simulink model "PSB_FPGAdesign8_model"  (R2021a)
settings: Solver=VariableStepAuto  StartTime=0.0  StopTime=3000  RelTol=1e-3
values from neighbouring files (symbols this model uses):
  n_channel = 1024    [PSB3_0_script.m]    (also in PSB_FPGAdesign8_script.m)
  parallel_factor = 4    [PSB3_0_script.m]    (also in PSB_FPGAdesign8_script.m)
libraries: xbsIndex_r4 x1089, xrbsSSR_Library x150, dspsrcs4 x48
(part 3 of 7)

== system PSB_FPGAdesign8_model/Baseband_odd_3 ==
  tvalid : Inport
  addr_r : Inport  Port=2
  addr_w : Inport  Port=3
  init_im_odd : Inport  Port=4
  init_re_odd : Inport  Port=5
  dphi_odd : Inport  Port=6
  we : Inport  Port=7
  AddSub1 : xbsIndex_r4/AddSub  mode=Addition  use_carryin=off  use_carryout=off  en=off  latency=2  precision=User Defined  arith_type=Unsigned  n_bits=16  bin_pt=0  quantization=Truncate  overflow=Wrap  use_behavioral_HDL=off  hw_selection=Fabric  pipelined=off  dbl_ovrd=off  block_type=addsub
  CORDIC 6.0 odd_1 : xbsIndex_r4/CORDIC 6.0   functional_selection=Rotate  architectural_configuration=Parallel  pipelining_mode=Optimal  data_format=SignedFraction  phase_format=Scaled_Radians  input_width=18  output_width=16  round_mode=Nearest_Even  iterations=16  precision=20  compensation_scaling=LUT_based  coarse_rotation=on  aclken=off  aresetn=off  out_tready=off  cartesian_has_tuser=off  cartesian_has_tlast=off  cartesian_tuser_width=1  phase_has_tuser=off  phase_has_tlast=off  phase_tuser_width=1  out_tlast_behv=Null  flow_control=NonBlocking  optimize_goal=Resources  trim_axipin_name=on  simulation_type=hybrid_sim  simulation_model=sysgen:cordic_v6_0  data_path_portlist={'s_axis_cartesian_tdata_imag', 's_axis_cartesian_tdata_real', 's_axis_phase_tdata_phase', 'm_axis_dout_tdata_imag', 'm_axis_dout_tdata_real', 'm_axis_dout_tdata_phase','m_axis_dout_tdata'}  ip_name=CORDIC  ip_version=6.0  dsptool_ready=true  ipcore_usecache=true  ipcore_useipmodelcache=true  wrapper_available=true  port_translation_map={ 'aclken' => 'en', 'aresetn' => 'rst' }  block_type=cordic_v6_0
      settings: infoedit=CORDIC 6.0
  Constant10 : xbsIndex_r4/Constant  const=0  gui_display_data_type=Fixed-point  arith_type=Signed (2's comp)  n_bits=18  bin_pt=16  preci_type=Single  exp_width=8  frac_width=24  explicit_period=on  period=1  equ=P=C  opselect=C  inp2=PCIN>>17  opr=+  inp1=P  carry=CIN  dbl_ovrd=off  block_type=constant
  Constant11 : xbsIndex_r4/Constant  const=1  gui_display_data_type=Boolean  arith_type=Boolean  n_bits=16  bin_pt=14  preci_type=Single  exp_width=8  frac_width=24  explicit_period=on  period=1  equ=P=C  opselect=C  inp2=PCIN>>17  opr=+  inp1=P  carry=CIN  dbl_ovrd=off  block_type=constant
  Constant12 : xbsIndex_r4/Constant  const=0  gui_display_data_type=Fixed-point  arith_type=Signed (2's comp)  n_bits=18  bin_pt=16  preci_type=Single  exp_width=8  frac_width=24  explicit_period=on  period=1  equ=P=C  opselect=C  inp2=PCIN>>17  opr=+  inp1=P  carry=CIN  dbl_ovrd=off  block_type=constant
  Constant13 : xbsIndex_r4/Constant  const=0  gui_display_data_type=Fixed-point  arith_type=Unsigned  n_bits=16  bin_pt=0  preci_type=Single  exp_width=8  frac_width=24  explicit_period=on  period=1  equ=P=C  opselect=C  inp2=PCIN>>17  opr=+  inp1=P  carry=CIN  dbl_ovrd=off  block_type=constant
  Constant4 : xbsIndex_r4/Constant  const=0  gui_display_data_type=Boolean  arith_type=Boolean  n_bits=16  bin_pt=14  preci_type=Single  exp_width=8  frac_width=24  explicit_period=on  period=1  equ=P=C  opselect=C  inp2=PCIN>>17  opr=+  inp1=P  carry=CIN  dbl_ovrd=off  block_type=constant
  Constant5 : xbsIndex_r4/Constant  const=0  gui_display_data_type=Boolean  arith_type=Boolean  n_bits=16  bin_pt=14  preci_type=Single  exp_width=8  frac_width=24  explicit_period=on  period=1  equ=P=C  opselect=C  inp2=PCIN>>17  opr=+  inp1=P  carry=CIN  dbl_ovrd=off  block_type=constant
  Constant9 : xbsIndex_r4/Constant  const=0  gui_display_data_type=Boolean  arith_type=Boolean  n_bits=16  bin_pt=14  preci_type=Single  exp_width=8  frac_width=24  explicit_period=on  period=1  equ=P=C  opselect=C  inp2=PCIN>>17  opr=+  inp1=P  carry=CIN  dbl_ovrd=off  block_type=constant
  Convert1 : xbsIndex_r4/Convert  gui_display_data_type=Fixed-point  arith_type="Signed  (2's comp)"  n_bits=18  bin_pt=15  float_type=Single  exp_bits=8  fraction_bits=24  quantization=Truncate  overflow=Wrap  en=off  latency=0  pipeline=off  dbl_ovrd=off  block_type=convert
  DPRAM_dphi_odd_3 : xbsIndex_r4/Dual Port RAM  depth=n_channel/parallel_factor  initVector=dphi_uint16_odd_3  distributed_mem=Block RAM  init_a=0  init_b=0  rst_a=off  rst_b=off  en_a=off  en_b=off  latency=1  write_mode_A=Read Before Write  write_mode_B=Read Before Write  optimize=Area  dbl_ovrd=off  simulation_type=fast_sim  block_type=dpram
  DPRAM_init_im_odd_3 : xbsIndex_r4/Dual Port RAM  depth=n_channel/parallel_factor  initVector=init_im_odd_3  distributed_mem=Block RAM  init_a=0  init_b=0  rst_a=off  rst_b=off  en_a=off  en_b=off  latency=1  write_mode_A=Read Before Write  write_mode_B=Read Before Write  optimize=Area  dbl_ovrd=off  simulation_type=fast_sim  block_type=dpram
  DPRAM_init_re_odd_3 : xbsIndex_r4/Dual Port RAM  depth=n_channel/parallel_factor  initVector=init_re_odd_3  distributed_mem=Block RAM  init_a=0  init_b=0  rst_a=off  rst_b=off  en_a=off  en_b=off  latency=1  write_mode_A=Read Before Write  write_mode_B=Read Before Write  optimize=Area  dbl_ovrd=off  simulation_type=fast_sim  block_type=dpram
  Delay8 : xbsIndex_r4/Delay  rst=off  infoeditControl=Selection of Reset will increase slice count due to use of real FFs and instead of SRLs  en=off  latency=n_channel/parallel_factor-2-1  reg_retiming=off  dbl_ovrd=off  block_type=delay
  FIFO1 : xbsIndex_r4/FIFO  mem_type=Block RAM  performance_options=Standard_FIFO  embedded_registers=off  depth=1K  percent_nbits=1  rst=off  rst_latency=2  en=off  use_dcount=off  use_percent_full_port=off  use_almost_empty=off  almost_empty_thresh=2  use_almost_full=off  use_rd_rst_busy=off  use_wr_rst_busy=off  almost_full_thresh=14  explicit_period=off  dbl_ovrd=off  simulation_type=fast_sim  block_type=fifo
  Reinterpret1 : xbsIndex_r4/Reinterpret  force_arith_type=on  arith_type="Signed  (2's comp)"  force_bin_pt=on  bin_pt=15  block_type=reinterpret
  Terminator{6..8,10,12} (5 alike) : Terminator
  delayCounter1 : Subsystem
  delay_count : Outport
  out_im : Outport  Port=2
  out_re : Outport  Port=3
  out_tvalid : Outport  Port=4
  wires:
  CORDIC 6.0 odd_1/1 -> out_tvalid/1, delayCounter1/2(edge2)
  CORDIC 6.0 odd_1/2 -> out_im/1
  init_im_odd/1 -> DPRAM_init_im_odd_3/5
  dphi_odd/1 -> DPRAM_dphi_odd_3/5
  FIFO1/2 -> Terminator12/1
  Reinterpret1/1 -> Convert1/1
  DPRAM_dphi_odd_3/1 -> AddSub1/1
  delayCounter1/1(delay) -> delay_count/1
  Constant9/1 -> DPRAM_dphi_odd_3/3
  addr_w/1 -> DPRAM_dphi_odd_3/4, DPRAM_init_re_odd_3/4, DPRAM_init_im_odd_3/4
  AddSub1/1 -> FIFO1/1
  Convert1/1 -> CORDIC 6.0 odd_1/5
  DPRAM_init_im_odd_3/2 -> Terminator7/1
  DPRAM_init_re_odd_3/2 -> Terminator8/1
  Constant11/1 -> FIFO1/2, Delay8/1
  DPRAM_init_re_odd_3/1 -> CORDIC 6.0 odd_1/3
  Constant4/1 -> DPRAM_init_im_odd_3/3
  Constant5/1 -> DPRAM_init_re_odd_3/3
  Constant10/1 -> DPRAM_init_im_odd_3/2
  FIFO1/1 -> AddSub1/2, Reinterpret1/1
  CORDIC 6.0 odd_1/3 -> out_re/1
  DPRAM_dphi_odd_3/2 -> Terminator10/1
  DPRAM_init_im_odd_3/1 -> CORDIC 6.0 odd_1/2
  Constant13/1 -> DPRAM_dphi_odd_3/2
  FIFO1/3 -> Terminator6/1
  addr_r/1 -> DPRAM_dphi_odd_3/1, DPRAM_init_re_odd_3/1, DPRAM_init_im_odd_3/1
  init_re_odd/1 -> DPRAM_init_re_odd_3/5
  Constant12/1 -> DPRAM_init_re_odd_3/2
  we/1 -> DPRAM_dphi_odd_3/6, DPRAM_init_re_odd_3/6, DPRAM_init_im_odd_3/6
  tvalid/1 -> delayCounter1/1(edge1), CORDIC 6.0 odd_1/4, CORDIC 6.0 odd_1/1
  Delay8/1 -> FIFO1/3

== system PSB_FPGAdesign8_model/Baseband_odd_4 ==
  tvalid : Inport
  addr_r : Inport  Port=2
  addr_w : Inport  Port=3
  init_im_odd_2 : Inport  Port=4
  init_re_odd_2 : Inport  Port=5
  dphi_odd_2 : Inport  Port=6
  we : Inport  Port=7
  AddSub1 : xbsIndex_r4/AddSub  mode=Addition  use_carryin=off  use_carryout=off  en=off  latency=2  precision=User Defined  arith_type=Unsigned  n_bits=16  bin_pt=0  quantization=Truncate  overflow=Wrap  use_behavioral_HDL=off  hw_selection=Fabric  pipelined=off  dbl_ovrd=off  block_type=addsub
  CORDIC 6.0 odd_2 : xbsIndex_r4/CORDIC 6.0   functional_selection=Rotate  architectural_configuration=Parallel  pipelining_mode=Optimal  data_format=SignedFraction  phase_format=Scaled_Radians  input_width=18  output_width=16  round_mode=Nearest_Even  iterations=16  precision=20  compensation_scaling=LUT_based  coarse_rotation=on  aclken=off  aresetn=off  out_tready=off  cartesian_has_tuser=off  cartesian_has_tlast=off  cartesian_tuser_width=1  phase_has_tuser=off  phase_has_tlast=off  phase_tuser_width=1  out_tlast_behv=Null  flow_control=NonBlocking  optimize_goal=Resources  trim_axipin_name=on  simulation_type=hybrid_sim  simulation_model=sysgen:cordic_v6_0  data_path_portlist={'s_axis_cartesian_tdata_imag', 's_axis_cartesian_tdata_real', 's_axis_phase_tdata_phase', 'm_axis_dout_tdata_imag', 'm_axis_dout_tdata_real', 'm_axis_dout_tdata_phase','m_axis_dout_tdata'}  ip_name=CORDIC  ip_version=6.0  dsptool_ready=true  ipcore_usecache=true  ipcore_useipmodelcache=true  wrapper_available=true  port_translation_map={ 'aclken' => 'en', 'aresetn' => 'rst' }  block_type=cordic_v6_0
      settings: infoedit=CORDIC 6.0
  Constant10 : xbsIndex_r4/Constant  const=0  gui_display_data_type=Fixed-point  arith_type=Signed (2's comp)  n_bits=18  bin_pt=16  preci_type=Single  exp_width=8  frac_width=24  explicit_period=on  period=1  equ=P=C  opselect=C  inp2=PCIN>>17  opr=+  inp1=P  carry=CIN  dbl_ovrd=off  block_type=constant
  Constant11 : xbsIndex_r4/Constant  const=1  gui_display_data_type=Boolean  arith_type=Boolean  n_bits=16  bin_pt=14  preci_type=Single  exp_width=8  frac_width=24  explicit_period=on  period=1  equ=P=C  opselect=C  inp2=PCIN>>17  opr=+  inp1=P  carry=CIN  dbl_ovrd=off  block_type=constant
  Constant12 : xbsIndex_r4/Constant  const=0  gui_display_data_type=Fixed-point  arith_type=Signed (2's comp)  n_bits=18  bin_pt=16  preci_type=Single  exp_width=8  frac_width=24  explicit_period=on  period=1  equ=P=C  opselect=C  inp2=PCIN>>17  opr=+  inp1=P  carry=CIN  dbl_ovrd=off  block_type=constant
  Constant13 : xbsIndex_r4/Constant  const=0  gui_display_data_type=Fixed-point  arith_type=Unsigned  n_bits=16  bin_pt=0  preci_type=Single  exp_width=8  frac_width=24  explicit_period=on  period=1  equ=P=C  opselect=C  inp2=PCIN>>17  opr=+  inp1=P  carry=CIN  dbl_ovrd=off  block_type=constant
  Constant4 : xbsIndex_r4/Constant  const=0  gui_display_data_type=Boolean  arith_type=Boolean  n_bits=16  bin_pt=14  preci_type=Single  exp_width=8  frac_width=24  explicit_period=on  period=1  equ=P=C  opselect=C  inp2=PCIN>>17  opr=+  inp1=P  carry=CIN  dbl_ovrd=off  block_type=constant
  Constant5 : xbsIndex_r4/Constant  const=0  gui_display_data_type=Boolean  arith_type=Boolean  n_bits=16  bin_pt=14  preci_type=Single  exp_width=8  frac_width=24  explicit_period=on  period=1  equ=P=C  opselect=C  inp2=PCIN>>17  opr=+  inp1=P  carry=CIN  dbl_ovrd=off  block_type=constant
  Constant9 : xbsIndex_r4/Constant  const=0  gui_display_data_type=Boolean  arith_type=Boolean  n_bits=16  bin_pt=14  preci_type=Single  exp_width=8  frac_width=24  explicit_period=on  period=1  equ=P=C  opselect=C  inp2=PCIN>>17  opr=+  inp1=P  carry=CIN  dbl_ovrd=off  block_type=constant
  Convert1 : xbsIndex_r4/Convert  gui_display_data_type=Fixed-point  arith_type="Signed  (2's comp)"  n_bits=18  bin_pt=15  float_type=Single  exp_bits=8  fraction_bits=24  quantization=Truncate  overflow=Wrap  en=off  latency=0  pipeline=off  dbl_ovrd=off  block_type=convert
  DPRAM_dphi_odd_4 : xbsIndex_r4/Dual Port RAM  depth=n_channel/parallel_factor  initVector=dphi_uint16_odd_4  distributed_mem=Block RAM  init_a=0  init_b=0  rst_a=off  rst_b=off  en_a=off  en_b=off  latency=1  write_mode_A=Read Before Write  write_mode_B=Read Before Write  optimize=Area  dbl_ovrd=off  simulation_type=fast_sim  block_type=dpram
  DPRAM_init_im_odd_4 : xbsIndex_r4/Dual Port RAM  depth=n_channel/parallel_factor  initVector=init_im_odd_4  distributed_mem=Block RAM  init_a=0  init_b=0  rst_a=off  rst_b=off  en_a=off  en_b=off  latency=1  write_mode_A=Read Before Write  write_mode_B=Read Before Write  optimize=Area  dbl_ovrd=off  simulation_type=fast_sim  block_type=dpram
  DPRAM_init_re_odd_4 : xbsIndex_r4/Dual Port RAM  depth=n_channel/parallel_factor  initVector=init_re_odd_4  distributed_mem=Block RAM  init_a=0  init_b=0  rst_a=off  rst_b=off  en_a=off  en_b=off  latency=1  write_mode_A=Read Before Write  write_mode_B=Read Before Write  optimize=Area  dbl_ovrd=off  simulation_type=fast_sim  block_type=dpram
  Delay8 : xbsIndex_r4/Delay  rst=off  infoeditControl=Selection of Reset will increase slice count due to use of real FFs and instead of SRLs  en=off  latency=n_channel/parallel_factor-2-1  reg_retiming=off  dbl_ovrd=off  block_type=delay
  FIFO1 : xbsIndex_r4/FIFO  mem_type=Block RAM  performance_options=Standard_FIFO  embedded_registers=off  depth=1K  percent_nbits=1  rst=off  rst_latency=2  en=off  use_dcount=off  use_percent_full_port=off  use_almost_empty=off  almost_empty_thresh=2  use_almost_full=off  use_rd_rst_busy=off  use_wr_rst_busy=off  almost_full_thresh=14  explicit_period=off  dbl_ovrd=off  simulation_type=fast_sim  block_type=fifo
  Reinterpret1 : xbsIndex_r4/Reinterpret  force_arith_type=on  arith_type="Signed  (2's comp)"  force_bin_pt=on  bin_pt=15  block_type=reinterpret
  Terminator{6..8,10,12} (5 alike) : Terminator
  delayCounter_odd_2 : Subsystem
  delay_count : Outport
  out_im : Outport  Port=2
  out_re : Outport  Port=3
  out_tvalid : Outport  Port=4
  wires:
  CORDIC 6.0 odd_2/1 -> out_tvalid/1, delayCounter_odd_2/2(edge2)
  Delay8/1 -> FIFO1/3
  tvalid/1 -> CORDIC 6.0 odd_2/1, CORDIC 6.0 odd_2/4, delayCounter_odd_2/1(edge1)
  we/1 -> DPRAM_init_im_odd_4/6, DPRAM_init_re_odd_4/6, DPRAM_dphi_odd_4/6
  Constant12/1 -> DPRAM_init_re_odd_4/2
  init_re_odd_2/1 -> DPRAM_init_re_odd_4/5
  addr_r/1 -> DPRAM_init_im_odd_4/1, DPRAM_init_re_odd_4/1, DPRAM_dphi_odd_4/1
  FIFO1/3 -> Terminator6/1
  Constant13/1 -> DPRAM_dphi_odd_4/2
  DPRAM_init_im_odd_4/1 -> CORDIC 6.0 odd_2/2
  DPRAM_dphi_odd_4/2 -> Terminator10/1
  CORDIC 6.0 odd_2/3 -> out_re/1
  FIFO1/1 -> Reinterpret1/1, AddSub1/2
  Constant10/1 -> DPRAM_init_im_odd_4/2
  Constant5/1 -> DPRAM_init_re_odd_4/3
  Constant4/1 -> DPRAM_init_im_odd_4/3
  DPRAM_init_re_odd_4/1 -> CORDIC 6.0 odd_2/3
  Constant11/1 -> Delay8/1, FIFO1/2
  DPRAM_init_re_odd_4/2 -> Terminator8/1
  DPRAM_init_im_odd_4/2 -> Terminator7/1
  Convert1/1 -> CORDIC 6.0 odd_2/5
  AddSub1/1 -> FIFO1/1
  addr_w/1 -> DPRAM_init_im_odd_4/4, DPRAM_init_re_odd_4/4, DPRAM_dphi_odd_4/4
  Constant9/1 -> DPRAM_dphi_odd_4/3
  delayCounter_odd_2/1(delay) -> delay_count/1
  DPRAM_dphi_odd_4/1 -> AddSub1/1
  Reinterpret1/1 -> Convert1/1
  FIFO1/2 -> Terminator12/1
  dphi_odd_2/1 -> DPRAM_dphi_odd_4/5
  init_im_odd_2/1 -> DPRAM_init_im_odd_4/5
  CORDIC 6.0 odd_2/2 -> out_im/1

== system PSB_FPGAdesign8_model/FIR_Coeff_1 ==
  Enable : EnablePort  StatesWhenEnabling=reset
  FIR_Coeff : dspsrcs4/Signal From Workspace  X=win_coeffs_reshaped_simulink_1  Ts=1  nsamps=1  OutputAfterFinalValue=Cyclic repetition  ignoreOrWarnInputAndFrameLengths=off  OutputFrames=off
  Outport : Outport
  wires:
  FIR_Coeff/1 -> Outport/1

== system PSB_FPGAdesign8_model/FIR_Coeff_2 ==
  Enable : EnablePort  StatesWhenEnabling=reset
  FIR_Coeff : dspsrcs4/Signal From Workspace  X=win_coeffs_reshaped_simulink_2  Ts=1  nsamps=1  OutputAfterFinalValue=Cyclic repetition  ignoreOrWarnInputAndFrameLengths=off  OutputFrames=off
  Outport : Outport
  wires:
  FIR_Coeff/1 -> Outport/1

== system PSB_FPGAdesign8_model/FIR_Coeff_3 ==
  Enable : EnablePort  StatesWhenEnabling=reset
  FIR_Coeff : dspsrcs4/Signal From Workspace  X=win_coeffs_reshaped_simulink_3  Ts=1  nsamps=1  OutputAfterFinalValue=Cyclic repetition  ignoreOrWarnInputAndFrameLengths=off  OutputFrames=off
  Outport : Outport
  wires:
  FIR_Coeff/1 -> Outport/1

== system PSB_FPGAdesign8_model/FIR_Coeff_4 ==
  Enable : EnablePort  StatesWhenEnabling=reset
  FIR_Coeff : dspsrcs4/Signal From Workspace  X=win_coeffs_reshaped_simulink_4  Ts=1  nsamps=1  OutputAfterFinalValue=Cyclic repetition  ignoreOrWarnInputAndFrameLengths=off  OutputFrames=off
  Outport : Outport
  wires:
  FIR_Coeff/1 -> Outport/1

== system PSB_FPGAdesign8_model/MemContents ==
  Enable : EnablePort
  w_addr : dspsrcs4/Signal From Workspace  X=[0:511]  Ts=1  nsamps=1  OutputAfterFinalValue=Setting to zero  ignoreOrWarnInputAndFrameLengths=on  OutputFrames=off
  w_dphi : dspsrcs4/Signal From Workspace  X=dphi_uint16_even_1  Ts=1  nsamps=1  OutputAfterFinalValue=Setting to zero  ignoreOrWarnInputAndFrameLengths=on  OutputFrames=off
  w_init_im : dspsrcs4/Signal From Workspace  X=init_im_even_1  Ts=1  nsamps=1  OutputAfterFinalValue=Setting to zero  ignoreOrWarnInputAndFrameLengths=on  OutputFrames=off
  w_init_re : dspsrcs4/Signal From Workspace  X=init_re_even_1  Ts=1  nsamps=1  OutputAfterFinalValue=Setting to zero  ignoreOrWarnInputAndFrameLengths=on  OutputFrames=off
  addr : Outport
  im : Outport  Port=2
  re : Outport  Port=3
  dp : Outport  Port=4
  wires:
  w_dphi/1 -> dp/1
  w_init_re/1 -> re/1
  w_init_im/1 -> im/1
  w_addr/1 -> addr/1

== system PSB_FPGAdesign8_model/MemContents1 ==
  Enable : EnablePort
  w_addr : dspsrcs4/Signal From Workspace  X=[0:511]  Ts=1  nsamps=1  OutputAfterFinalValue=Setting to zero  ignoreOrWarnInputAndFrameLengths=on  OutputFrames=off
  w_dphi : dspsrcs4/Signal From Workspace  X=dphi_uint16_odd_1  Ts=1  nsamps=1  OutputAfterFinalValue=Setting to zero  ignoreOrWarnInputAndFrameLengths=on  OutputFrames=off
  w_init_im : dspsrcs4/Signal From Workspace  X=init_im_odd_1  Ts=1  nsamps=1  OutputAfterFinalValue=Setting to zero  ignoreOrWarnInputAndFrameLengths=on  OutputFrames=off
  w_init_re : dspsrcs4/Signal From Workspace  X=init_re_odd_1  Ts=1  nsamps=1  OutputAfterFinalValue=Setting to zero  ignoreOrWarnInputAndFrameLengths=on  OutputFrames=off
  addr : Outport
  im : Outport  Port=2
  re : Outport  Port=3
  dp : Outport  Port=4
  wires:
  w_dphi/1 -> dp/1  "TL_dphi"
  w_init_re/1 -> re/1  "TL_init_re"
  w_init_im/1 -> im/1  "TL_init_im"
  w_addr/1 -> addr/1  "w_addr"

== system PSB_FPGAdesign8_model/MemContents2 ==
  Enable : EnablePort
  w_addr : dspsrcs4/Signal From Workspace  X=[0:511]  Ts=1  nsamps=1  OutputAfterFinalValue=Setting to zero  ignoreOrWarnInputAndFrameLengths=on  OutputFrames=off
  w_dphi : dspsrcs4/Signal From Workspace  X=dphi_uint16_even_2  Ts=1  nsamps=1  OutputAfterFinalValue=Setting to zero  ignoreOrWarnInputAndFrameLengths=on  OutputFrames=off
  w_init_im : dspsrcs4/Signal From Workspace  X=init_im_even_2  Ts=1  nsamps=1  OutputAfterFinalValue=Setting to zero  ignoreOrWarnInputAndFrameLengths=on  OutputFrames=off
  w_init_re : dspsrcs4/Signal From Workspace  X=init_re_even_2  Ts=1  nsamps=1  OutputAfterFinalValue=Setting to zero  ignoreOrWarnInputAndFrameLengths=on  OutputFrames=off
  addr : Outport
  im : Outport  Port=2
  re : Outport  Port=3
  dp : Outport  Port=4
  wires:
  w_addr/1 -> addr/1
  w_init_im/1 -> im/1
  w_init_re/1 -> re/1
  w_dphi/1 -> dp/1

== system PSB_FPGAdesign8_model/MemContents3 ==
  Enable : EnablePort
  w_addr : dspsrcs4/Signal From Workspace  X=[0:511]  Ts=1  nsamps=1  OutputAfterFinalValue=Setting to zero  ignoreOrWarnInputAndFrameLengths=on  OutputFrames=off
  w_dphi : dspsrcs4/Signal From Workspace  X=dphi_uint16_odd_2  Ts=1  nsamps=1  OutputAfterFinalValue=Setting to zero  ignoreOrWarnInputAndFrameLengths=on  OutputFrames=off
  w_init_im : dspsrcs4/Signal From Workspace  X=init_im_odd_2  Ts=1  nsamps=1  OutputAfterFinalValue=Setting to zero  ignoreOrWarnInputAndFrameLengths=on  OutputFrames=off
  w_init_re : dspsrcs4/Signal From Workspace  X=init_re_odd_2  Ts=1  nsamps=1  OutputAfterFinalValue=Setting to zero  ignoreOrWarnInputAndFrameLengths=on  OutputFrames=off
  addr : Outport
  im : Outport  Port=2
  re : Outport  Port=3
  dp : Outport  Port=4
  wires:
  w_addr/1 -> addr/1  "w_addr"
  w_init_im/1 -> im/1  "TL_init_im"
  w_init_re/1 -> re/1  "TL_init_re"
  w_dphi/1 -> dp/1  "TL_dphi"

== system PSB_FPGAdesign8_model/MemContents4 ==
  Enable : EnablePort
  w_addr : dspsrcs4/Signal From Workspace  X=[0:255]  Ts=1  nsamps=1  OutputAfterFinalValue=Setting to zero  ignoreOrWarnInputAndFrameLengths=on  OutputFrames=off
  w_dphi : dspsrcs4/Signal From Workspace  X=dphi_uint16_even_3  Ts=1  nsamps=1  OutputAfterFinalValue=Setting to zero  ignoreOrWarnInputAndFrameLengths=on  OutputFrames=off
  w_init_im : dspsrcs4/Signal From Workspace  X=init_im_even_3  Ts=1  nsamps=1  OutputAfterFinalValue=Setting to zero  ignoreOrWarnInputAndFrameLengths=on  OutputFrames=off
  w_init_re : dspsrcs4/Signal From Workspace  X=init_re_even_3  Ts=1  nsamps=1  OutputAfterFinalValue=Setting to zero  ignoreOrWarnInputAndFrameLengths=on  OutputFrames=off
  addr : Outport
  im : Outport  Port=2
  re : Outport  Port=3
  dp : Outport  Port=4
  wires:
  w_addr/1 -> addr/1
  w_init_im/1 -> im/1
  w_init_re/1 -> re/1
  w_dphi/1 -> dp/1

== system PSB_FPGAdesign8_model/MemContents5 ==
  Enable : EnablePort
  w_addr : dspsrcs4/Signal From Workspace  X=[0:255]  Ts=1  nsamps=1  OutputAfterFinalValue=Setting to zero  ignoreOrWarnInputAndFrameLengths=on  OutputFrames=off
  w_dphi : dspsrcs4/Signal From Workspace  X=dphi_uint16_odd_3  Ts=1  nsamps=1  OutputAfterFinalValue=Setting to zero  ignoreOrWarnInputAndFrameLengths=on  OutputFrames=off
  w_init_im : dspsrcs4/Signal From Workspace  X=init_im_odd_3  Ts=1  nsamps=1  OutputAfterFinalValue=Setting to zero  ignoreOrWarnInputAndFrameLengths=on  OutputFrames=off
  w_init_re : dspsrcs4/Signal From Workspace  X=init_re_odd_3  Ts=1  nsamps=1  OutputAfterFinalValue=Setting to zero  ignoreOrWarnInputAndFrameLengths=on  OutputFrames=off
  addr : Outport
  im : Outport  Port=2
  re : Outport  Port=3
  dp : Outport  Port=4
  wires:
  w_addr/1 -> addr/1  "w_addr"
  w_init_im/1 -> im/1  "TL_init_im"
  w_init_re/1 -> re/1  "TL_init_re"
  w_dphi/1 -> dp/1  "TL_dphi"

== system PSB_FPGAdesign8_model/MemContents6 ==
  Enable : EnablePort
  w_addr : dspsrcs4/Signal From Workspace  X=[0:255]  Ts=1  nsamps=1  OutputAfterFinalValue=Setting to zero  ignoreOrWarnInputAndFrameLengths=on  OutputFrames=off
  w_dphi : dspsrcs4/Signal From Workspace  X=dphi_uint16_even_4  Ts=1  nsamps=1  OutputAfterFinalValue=Setting to zero  ignoreOrWarnInputAndFrameLengths=on  OutputFrames=off
  w_init_im : dspsrcs4/Signal From Workspace  X=init_im_even_4  Ts=1  nsamps=1  OutputAfterFinalValue=Setting to zero  ignoreOrWarnInputAndFrameLengths=on  OutputFrames=off
  w_init_re : dspsrcs4/Signal From Workspace  X=init_re_even_4  Ts=1  nsamps=1  OutputAfterFinalValue=Setting to zero  ignoreOrWarnInputAndFrameLengths=on  OutputFrames=off
  addr : Outport
  im : Outport  Port=2
  re : Outport  Port=3
  dp : Outport  Port=4
  wires:
  w_dphi/1 -> dp/1
  w_init_re/1 -> re/1
  w_init_im/1 -> im/1
  w_addr/1 -> addr/1

== system PSB_FPGAdesign8_model/MemContents7 ==
  Enable : EnablePort
  w_addr : dspsrcs4/Signal From Workspace  X=[0:255]  Ts=1  nsamps=1  OutputAfterFinalValue=Setting to zero  ignoreOrWarnInputAndFrameLengths=on  OutputFrames=off
  w_dphi : dspsrcs4/Signal From Workspace  X=dphi_uint16_odd_4  Ts=1  nsamps=1  OutputAfterFinalValue=Setting to zero  ignoreOrWarnInputAndFrameLengths=on  OutputFrames=off
  w_init_im : dspsrcs4/Signal From Workspace  X=init_im_odd_4  Ts=1  nsamps=1  OutputAfterFinalValue=Setting to zero  ignoreOrWarnInputAndFrameLengths=on  OutputFrames=off
  w_init_re : dspsrcs4/Signal From Workspace  X=init_re_odd_4  Ts=1  nsamps=1  OutputAfterFinalValue=Setting to zero  ignoreOrWarnInputAndFrameLengths=on  OutputFrames=off
  addr : Outport
  im : Outport  Port=2
  re : Outport  Port=3
  dp : Outport  Port=4
  wires:
  w_dphi/1 -> dp/1  "TL_dphi"
  w_init_re/1 -> re/1  "TL_init_re"
  w_init_im/1 -> im/1  "TL_init_im"
  w_addr/1 -> addr/1  "w_addr"

== system PSB_FPGAdesign8_model/Overflow Detector add_im_1 ==
  rst : Inport
  A : Inport  Port=2
  B : Inport  Port=3
  S : Inport  Port=4
  Constant17 : xbsIndex_r4/Constant  const=1  gui_display_data_type=Boolean  arith_type=Boolean  n_bits=16  bin_pt=14  preci_type=Single  exp_width=8  frac_width=24  explicit_period=on  period=1  equ=P=C  opselect=C  inp2=PCIN>>17  opr=+  inp1=P  carry=CIN  dbl_ovrd=off  block_type=constant
  Convert : xbsIndex_r4/Convert  gui_display_data_type=Boolean  arith_type=Boolean  n_bits=16  bin_pt=14  float_type=Single  exp_bits=8  fraction_bits=24  quantization=Truncate  overflow=Wrap  en=off  latency=1  pipeline=off  dbl_ovrd=off  block_type=convert
  Expression : xbsIndex_r4/Expression  expression=(A & B & ~S) | (~A & ~B & S)  align_bp=off  en=off  latency=1  precision=User Defined  arith_type=Unsigned  n_bits=1  bin_pt=0  dbl_ovrd=off  block_type=expr
  Register : xbsIndex_r4/Register  init=0  rst=on  en=on  dbl_ovrd=off  block_type=register
  Vector Delay : xrbsSSR_Library/Vector Delay  sg_latency=2  infoeditControl=Selection of Reset will increase slice count due to use of real FFs and instead of SRLs  en=off  vectorize_en=off  rst=off  reg_retiming=off  block_type=delay_ssr  dbl_ovrd=off  sg_ssr=16  sg_ssr_prev=16  sg_ssr_name=vect_delay
      settings: SourceProductName=Xilinx SSR Blockset
  Vector Delay1 : xrbsSSR_Library/Vector Delay  sg_latency=2  infoeditControl=Selection of Reset will increase slice count due to use of real FFs and instead of SRLs  en=off  vectorize_en=off  rst=off  reg_retiming=off  block_type=delay_ssr  dbl_ovrd=off  sg_ssr=16  sg_ssr_prev=16  sg_ssr_name=vect_delay
      settings: SourceProductName=Xilinx SSR Blockset
  Vector Slice : xrbsSSR_Library/Vector Slice  nbits=1  sg_ssr=16  sg_ssr_prev=16  boolean_output=on  mode=Upper Bit Location + Width  bit1=0  base1=MSB of Input  bit0=0  base0=LSB of Input  dbl_ovrd=off  block_type=slice_ssr  sg_ssr_name=vect_slice
      settings: SourceProductName=Xilinx SSR Blockset  infoedit="The Vector Slice block supports input of vector types. Extracts a given range of bits from each sample of input vector and presents it at the output.  The output type is ordinarily unsigned with binary point at zero, but can be Boolean when the slice is one bit wide.<br><br>Hardware notes: In hardware this block costs nothing."
  Vector Slice1 : xrbsSSR_Library/Vector Slice  nbits=1  sg_ssr=16  sg_ssr_prev=16  boolean_output=on  mode=Upper Bit Location + Width  bit1=0  base1=MSB of Input  bit0=0  base0=LSB of Input  dbl_ovrd=off  block_type=slice_ssr  sg_ssr_name=vect_slice
      settings: SourceProductName=Xilinx SSR Blockset  infoedit="The Vector Slice block supports input of vector types. Extracts a given range of bits from each sample of input vector and presents it at the output.  The output type is ordinarily unsigned with binary point at zero, but can be Boolean when the slice is one bit wide.<br><br>Hardware notes: In hardware this block costs nothing."
  Vector Slice2 : xrbsSSR_Library/Vector Slice  nbits=1  sg_ssr=16  sg_ssr_prev=16  boolean_output=on  mode=Upper Bit Location + Width  bit1=0  base1=MSB of Input  bit0=0  base0=LSB of Input  dbl_ovrd=off  block_type=slice_ssr  sg_ssr_name=vect_slice
      settings: SourceProductName=Xilinx SSR Blockset  infoedit="The Vector Slice block supports input of vector types. Extracts a given range of bits from each sample of input vector and presents it at the output.  The output type is ordinarily unsigned with binary point at zero, but can be Boolean when the slice is one bit wide.<br><br>Hardware notes: In hardware this block costs nothing."
  Vector to Scalar : xrbsSSR_Library/Vector2Scalar  sg_ssr=16  sg_ssr_prev=16  sg_ssr_name=vect_Vector2Scalar  block_type=vector2scalar_ssr
      settings: SourceProductName=Xilinx SSR Blockset
  Vector to Scalar1 : xrbsSSR_Library/Vector2Scalar  sg_ssr=16  sg_ssr_prev=16  sg_ssr_name=vect_Vector2Scalar  block_type=vector2scalar_ssr
      settings: SourceProductName=Xilinx SSR Blockset
  Vector to Scalar2 : xrbsSSR_Library/Vector2Scalar  sg_ssr=16  sg_ssr_prev=16  sg_ssr_name=vect_Vector2Scalar  block_type=vector2scalar_ssr
      settings: SourceProductName=Xilinx SSR Blockset
  ov : Outport
  wires:
  Register/1 -> ov/1
  A/1 -> Vector Slice/1
  rst/1 -> Register/2
  Constant17/1 -> Register/1
  B/1 -> Vector Slice1/1
  S/1 -> Vector Slice2/1
  Vector Slice/1 -> Vector Delay/1
  Vector Slice1/1 -> Vector Delay1/1
  Vector Delay/1 -> Vector to Scalar/1
  Vector Delay1/1 -> Vector to Scalar1/1
  Vector Slice2/1 -> Vector to Scalar2/1
  Vector to Scalar/1 -> Expression/1
  Vector to Scalar1/1 -> Expression/2
  Vector to Scalar2/1 -> Expression/3
  Expression/1 -> Convert/1
  Convert/1 -> Register/3

== system PSB_FPGAdesign8_model/Overflow Detector add_im_2 ==
  rst : Inport
  A : Inport  Port=2
  B : Inport  Port=3
  S : Inport  Port=4
  Constant17 : xbsIndex_r4/Constant  const=1  gui_display_data_type=Boolean  arith_type=Boolean  n_bits=16  bin_pt=14  preci_type=Single  exp_width=8  frac_width=24  explicit_period=on  period=1  equ=P=C  opselect=C  inp2=PCIN>>17  opr=+  inp1=P  carry=CIN  dbl_ovrd=off  block_type=constant
  Convert : xbsIndex_r4/Convert  gui_display_data_type=Boolean  arith_type=Boolean  n_bits=16  bin_pt=14  float_type=Single  exp_bits=8  fraction_bits=24  quantization=Truncate  overflow=Wrap  en=off  latency=1  pipeline=off  dbl_ovrd=off  block_type=convert
  Expression : xbsIndex_r4/Expression  expression=(A & B & ~S) | (~A & ~B & S)  align_bp=off  en=off  latency=1  precision=User Defined  arith_type=Unsigned  n_bits=1  bin_pt=0  dbl_ovrd=off  block_type=expr
  Register : xbsIndex_r4/Register  init=0  rst=on  en=on  dbl_ovrd=off  block_type=register
  Vector Delay : xrbsSSR_Library/Vector Delay  sg_latency=2  infoeditControl=Selection of Reset will increase slice count due to use of real FFs and instead of SRLs  en=off  vectorize_en=off  rst=off  reg_retiming=off  block_type=delay_ssr  dbl_ovrd=off  sg_ssr=16  sg_ssr_prev=16  sg_ssr_name=vect_delay
      settings: SourceProductName=Xilinx SSR Blockset
  Vector Delay1 : xrbsSSR_Library/Vector Delay  sg_latency=2  infoeditControl=Selection of Reset will increase slice count due to use of real FFs and instead of SRLs  en=off  vectorize_en=off  rst=off  reg_retiming=off  block_type=delay_ssr  dbl_ovrd=off  sg_ssr=16  sg_ssr_prev=16  sg_ssr_name=vect_delay
      settings: SourceProductName=Xilinx SSR Blockset
  Vector Slice : xrbsSSR_Library/Vector Slice  nbits=1  sg_ssr=16  sg_ssr_prev=16  boolean_output=on  mode=Upper Bit Location + Width  bit1=0  base1=MSB of Input  bit0=0  base0=LSB of Input  dbl_ovrd=off  block_type=slice_ssr  sg_ssr_name=vect_slice
      settings: SourceProductName=Xilinx SSR Blockset  infoedit="The Vector Slice block supports input of vector types. Extracts a given range of bits from each sample of input vector and presents it at the output.  The output type is ordinarily unsigned with binary point at zero, but can be Boolean when the slice is one bit wide.<br><br>Hardware notes: In hardware this block costs nothing."
  Vector Slice1 : xrbsSSR_Library/Vector Slice  nbits=1  sg_ssr=16  sg_ssr_prev=16  boolean_output=on  mode=Upper Bit Location + Width  bit1=0  base1=MSB of Input  bit0=0  base0=LSB of Input  dbl_ovrd=off  block_type=slice_ssr  sg_ssr_name=vect_slice
      settings: SourceProductName=Xilinx SSR Blockset  infoedit="The Vector Slice block supports input of vector types. Extracts a given range of bits from each sample of input vector and presents it at the output.  The output type is ordinarily unsigned with binary point at zero, but can be Boolean when the slice is one bit wide.<br><br>Hardware notes: In hardware this block costs nothing."
  Vector Slice2 : xrbsSSR_Library/Vector Slice  nbits=1  sg_ssr=16  sg_ssr_prev=16  boolean_output=on  mode=Upper Bit Location + Width  bit1=0  base1=MSB of Input  bit0=0  base0=LSB of Input  dbl_ovrd=off  block_type=slice_ssr  sg_ssr_name=vect_slice
      settings: SourceProductName=Xilinx SSR Blockset  infoedit="The Vector Slice block supports input of vector types. Extracts a given range of bits from each sample of input vector and presents it at the output.  The output type is ordinarily unsigned with binary point at zero, but can be Boolean when the slice is one bit wide.<br><br>Hardware notes: In hardware this block costs nothing."
  Vector to Scalar : xrbsSSR_Library/Vector2Scalar  sg_ssr=16  sg_ssr_prev=16  sg_ssr_name=vect_Vector2Scalar  block_type=vector2scalar_ssr
      settings: SourceProductName=Xilinx SSR Blockset
  Vector to Scalar1 : xrbsSSR_Library/Vector2Scalar  sg_ssr=16  sg_ssr_prev=16  sg_ssr_name=vect_Vector2Scalar  block_type=vector2scalar_ssr
      settings: SourceProductName=Xilinx SSR Blockset
  Vector to Scalar2 : xrbsSSR_Library/Vector2Scalar  sg_ssr=16  sg_ssr_prev=16  sg_ssr_name=vect_Vector2Scalar  block_type=vector2scalar_ssr
      settings: SourceProductName=Xilinx SSR Blockset
  ov : Outport
  wires:
  Register/1 -> ov/1
  A/1 -> Vector Slice/1
  rst/1 -> Register/2
  Constant17/1 -> Register/1
  B/1 -> Vector Slice1/1
  S/1 -> Vector Slice2/1
  Vector Slice/1 -> Vector Delay/1
  Vector Slice1/1 -> Vector Delay1/1
  Vector Delay/1 -> Vector to Scalar/1
  Vector Delay1/1 -> Vector to Scalar1/1
  Vector Slice2/1 -> Vector to Scalar2/1
  Vector to Scalar/1 -> Expression/1
  Vector to Scalar1/1 -> Expression/2
  Vector to Scalar2/1 -> Expression/3
  Expression/1 -> Convert/1
  Convert/1 -> Register/3

== system PSB_FPGAdesign8_model/Overflow Detector add_im_3 ==
  rst : Inport
  A : Inport  Port=2
  B : Inport  Port=3
  S : Inport  Port=4
  Constant17 : xbsIndex_r4/Constant  const=1  gui_display_data_type=Boolean  arith_type=Boolean  n_bits=16  bin_pt=14  preci_type=Single  exp_width=8  frac_width=24  explicit_period=on  period=1  equ=P=C  opselect=C  inp2=PCIN>>17  opr=+  inp1=P  carry=CIN  dbl_ovrd=off  block_type=constant
  Convert : xbsIndex_r4/Convert  gui_display_data_type=Boolean  arith_type=Boolean  n_bits=16  bin_pt=14  float_type=Single  exp_bits=8  fraction_bits=24  quantization=Truncate  overflow=Wrap  en=off  latency=1  pipeline=off  dbl_ovrd=off  block_type=convert
  Expression : xbsIndex_r4/Expression  expression=(A & B & ~S) | (~A & ~B & S)  align_bp=off  en=off  latency=1  precision=User Defined  arith_type=Unsigned  n_bits=1  bin_pt=0  dbl_ovrd=off  block_type=expr
  Register : xbsIndex_r4/Register  init=0  rst=on  en=on  dbl_ovrd=off  block_type=register
  Vector Delay : xrbsSSR_Library/Vector Delay  sg_latency=2  infoeditControl=Selection of Reset will increase slice count due to use of real FFs and instead of SRLs  en=off  vectorize_en=off  rst=off  reg_retiming=off  block_type=delay_ssr  dbl_ovrd=off  sg_ssr=16  sg_ssr_prev=16  sg_ssr_name=vect_delay
      settings: SourceProductName=Xilinx SSR Blockset
  Vector Delay1 : xrbsSSR_Library/Vector Delay  sg_latency=2  infoeditControl=Selection of Reset will increase slice count due to use of real FFs and instead of SRLs  en=off  vectorize_en=off  rst=off  reg_retiming=off  block_type=delay_ssr  dbl_ovrd=off  sg_ssr=16  sg_ssr_prev=16  sg_ssr_name=vect_delay
      settings: SourceProductName=Xilinx SSR Blockset
  Vector Slice : xrbsSSR_Library/Vector Slice  nbits=1  sg_ssr=16  sg_ssr_prev=16  boolean_output=on  mode=Upper Bit Location + Width  bit1=0  base1=MSB of Input  bit0=0  base0=LSB of Input  dbl_ovrd=off  block_type=slice_ssr  sg_ssr_name=vect_slice
      settings: SourceProductName=Xilinx SSR Blockset  infoedit="The Vector Slice block supports input of vector types. Extracts a given range of bits from each sample of input vector and presents it at the output.  The output type is ordinarily unsigned with binary point at zero, but can be Boolean when the slice is one bit wide.<br><br>Hardware notes: In hardware this block costs nothing."
  Vector Slice1 : xrbsSSR_Library/Vector Slice  nbits=1  sg_ssr=16  sg_ssr_prev=16  boolean_output=on  mode=Upper Bit Location + Width  bit1=0  base1=MSB of Input  bit0=0  base0=LSB of Input  dbl_ovrd=off  block_type=slice_ssr  sg_ssr_name=vect_slice
      settings: SourceProductName=Xilinx SSR Blockset  infoedit="The Vector Slice block supports input of vector types. Extracts a given range of bits from each sample of input vector and presents it at the output.  The output type is ordinarily unsigned with binary point at zero, but can be Boolean when the slice is one bit wide.<br><br>Hardware notes: In hardware this block costs nothing."
  Vector Slice2 : xrbsSSR_Library/Vector Slice  nbits=1  sg_ssr=16  sg_ssr_prev=16  boolean_output=on  mode=Upper Bit Location + Width  bit1=0  base1=MSB of Input  bit0=0  base0=LSB of Input  dbl_ovrd=off  block_type=slice_ssr  sg_ssr_name=vect_slice
      settings: SourceProductName=Xilinx SSR Blockset  infoedit="The Vector Slice block supports input of vector types. Extracts a given range of bits from each sample of input vector and presents it at the output.  The output type is ordinarily unsigned with binary point at zero, but can be Boolean when the slice is one bit wide.<br><br>Hardware notes: In hardware this block costs nothing."
  Vector to Scalar : xrbsSSR_Library/Vector2Scalar  sg_ssr=16  sg_ssr_prev=16  sg_ssr_name=vect_Vector2Scalar  block_type=vector2scalar_ssr
      settings: SourceProductName=Xilinx SSR Blockset
  Vector to Scalar1 : xrbsSSR_Library/Vector2Scalar  sg_ssr=16  sg_ssr_prev=16  sg_ssr_name=vect_Vector2Scalar  block_type=vector2scalar_ssr
      settings: SourceProductName=Xilinx SSR Blockset
  Vector to Scalar2 : xrbsSSR_Library/Vector2Scalar  sg_ssr=16  sg_ssr_prev=16  sg_ssr_name=vect_Vector2Scalar  block_type=vector2scalar_ssr
      settings: SourceProductName=Xilinx SSR Blockset
  ov : Outport
  wires:
  Register/1 -> ov/1
  A/1 -> Vector Slice/1
  rst/1 -> Register/2
  Constant17/1 -> Register/1
  B/1 -> Vector Slice1/1
  S/1 -> Vector Slice2/1
  Vector Slice/1 -> Vector Delay/1
  Vector Slice1/1 -> Vector Delay1/1
  Vector Delay/1 -> Vector to Scalar/1
  Vector Delay1/1 -> Vector to Scalar1/1
  Vector Slice2/1 -> Vector to Scalar2/1
  Vector to Scalar/1 -> Expression/1
  Vector to Scalar1/1 -> Expression/2
  Vector to Scalar2/1 -> Expression/3
  Expression/1 -> Convert/1
  Convert/1 -> Register/3

== system PSB_FPGAdesign8_model/Overflow Detector add_im_4 ==
  rst : Inport
  A : Inport  Port=2
  B : Inport  Port=3
  S : Inport  Port=4
  Constant17 : xbsIndex_r4/Constant  const=1  gui_display_data_type=Boolean  arith_type=Boolean  n_bits=16  bin_pt=14  preci_type=Single  exp_width=8  frac_width=24  explicit_period=on  period=1  equ=P=C  opselect=C  inp2=PCIN>>17  opr=+  inp1=P  carry=CIN  dbl_ovrd=off  block_type=constant
  Convert : xbsIndex_r4/Convert  gui_display_data_type=Boolean  arith_type=Boolean  n_bits=16  bin_pt=14  float_type=Single  exp_bits=8  fraction_bits=24  quantization=Truncate  overflow=Wrap  en=off  latency=1  pipeline=off  dbl_ovrd=off  block_type=convert
  Expression : xbsIndex_r4/Expression  expression=(A & B & ~S) | (~A & ~B & S)  align_bp=off  en=off  latency=1  precision=User Defined  arith_type=Unsigned  n_bits=1  bin_pt=0  dbl_ovrd=off  block_type=expr
  Register : xbsIndex_r4/Register  init=0  rst=on  en=on  dbl_ovrd=off  block_type=register
  Vector Delay : xrbsSSR_Library/Vector Delay  sg_latency=2  infoeditControl=Selection of Reset will increase slice count due to use of real FFs and instead of SRLs  en=off  vectorize_en=off  rst=off  reg_retiming=off  block_type=delay_ssr  dbl_ovrd=off  sg_ssr=16  sg_ssr_prev=16  sg_ssr_name=vect_delay
      settings: SourceProductName=Xilinx SSR Blockset
  Vector Delay1 : xrbsSSR_Library/Vector Delay  sg_latency=2  infoeditControl=Selection of Reset will increase slice count due to use of real FFs and instead of SRLs  en=off  vectorize_en=off  rst=off  reg_retiming=off  block_type=delay_ssr  dbl_ovrd=off  sg_ssr=16  sg_ssr_prev=16  sg_ssr_name=vect_delay
      settings: SourceProductName=Xilinx SSR Blockset
  Vector Slice : xrbsSSR_Library/Vector Slice  nbits=1  sg_ssr=16  sg_ssr_prev=16  boolean_output=on  mode=Upper Bit Location + Width  bit1=0  base1=MSB of Input  bit0=0  base0=LSB of Input  dbl_ovrd=off  block_type=slice_ssr  sg_ssr_name=vect_slice
      settings: SourceProductName=Xilinx SSR Blockset  infoedit="The Vector Slice block supports input of vector types. Extracts a given range of bits from each sample of input vector and presents it at the output.  The output type is ordinarily unsigned with binary point at zero, but can be Boolean when the slice is one bit wide.<br><br>Hardware notes: In hardware this block costs nothing."
  Vector Slice1 : xrbsSSR_Library/Vector Slice  nbits=1  sg_ssr=16  sg_ssr_prev=16  boolean_output=on  mode=Upper Bit Location + Width  bit1=0  base1=MSB of Input  bit0=0  base0=LSB of Input  dbl_ovrd=off  block_type=slice_ssr  sg_ssr_name=vect_slice
      settings: SourceProductName=Xilinx SSR Blockset  infoedit="The Vector Slice block supports input of vector types. Extracts a given range of bits from each sample of input vector and presents it at the output.  The output type is ordinarily unsigned with binary point at zero, but can be Boolean when the slice is one bit wide.<br><br>Hardware notes: In hardware this block costs nothing."
  Vector Slice2 : xrbsSSR_Library/Vector Slice  nbits=1  sg_ssr=16  sg_ssr_prev=16  boolean_output=on  mode=Upper Bit Location + Width  bit1=0  base1=MSB of Input  bit0=0  base0=LSB of Input  dbl_ovrd=off  block_type=slice_ssr  sg_ssr_name=vect_slice
      settings: SourceProductName=Xilinx SSR Blockset  infoedit="The Vector Slice block supports input of vector types. Extracts a given range of bits from each sample of input vector and presents it at the output.  The output type is ordinarily unsigned with binary point at zero, but can be Boolean when the slice is one bit wide.<br><br>Hardware notes: In hardware this block costs nothing."
  Vector to Scalar : xrbsSSR_Library/Vector2Scalar  sg_ssr=16  sg_ssr_prev=16  sg_ssr_name=vect_Vector2Scalar  block_type=vector2scalar_ssr
      settings: SourceProductName=Xilinx SSR Blockset
  Vector to Scalar1 : xrbsSSR_Library/Vector2Scalar  sg_ssr=16  sg_ssr_prev=16  sg_ssr_name=vect_Vector2Scalar  block_type=vector2scalar_ssr
      settings: SourceProductName=Xilinx SSR Blockset
  Vector to Scalar2 : xrbsSSR_Library/Vector2Scalar  sg_ssr=16  sg_ssr_prev=16  sg_ssr_name=vect_Vector2Scalar  block_type=vector2scalar_ssr
      settings: SourceProductName=Xilinx SSR Blockset
  ov : Outport
  wires:
  Register/1 -> ov/1
  A/1 -> Vector Slice/1
  rst/1 -> Register/2
  Constant17/1 -> Register/1
  B/1 -> Vector Slice1/1
  S/1 -> Vector Slice2/1
  Vector Slice/1 -> Vector Delay/1
  Vector Slice1/1 -> Vector Delay1/1
  Vector Delay/1 -> Vector to Scalar/1
  Vector Delay1/1 -> Vector to Scalar1/1
  Vector Slice2/1 -> Vector to Scalar2/1
  Vector to Scalar/1 -> Expression/1
  Vector to Scalar1/1 -> Expression/2
  Vector to Scalar2/1 -> Expression/3
  Expression/1 -> Convert/1
  Convert/1 -> Register/3

== system PSB_FPGAdesign8_model/Overflow Detector add_re_1 ==
  rst : Inport
  A : Inport  Port=2
  B : Inport  Port=3
  S : Inport  Port=4
  Constant17 : xbsIndex_r4/Constant  const=1  gui_display_data_type=Boolean  arith_type=Boolean  n_bits=16  bin_pt=14  preci_type=Single  exp_width=8  frac_width=24  explicit_period=on  period=1  equ=P=C  opselect=C  inp2=PCIN>>17  opr=+  inp1=P  carry=CIN  dbl_ovrd=off  block_type=constant
  Convert : xbsIndex_r4/Convert  gui_display_data_type=Boolean  arith_type=Boolean  n_bits=16  bin_pt=14  float_type=Single  exp_bits=8  fraction_bits=24  quantization=Truncate  overflow=Wrap  en=off  latency=1  pipeline=off  dbl_ovrd=off  block_type=convert
  Expression : xbsIndex_r4/Expression  expression=(A & B & ~S) | (~A & ~B & S)  align_bp=off  en=off  latency=1  precision=User Defined  arith_type=Unsigned  n_bits=1  bin_pt=0  dbl_ovrd=off  block_type=expr
  Register : xbsIndex_r4/Register  init=0  rst=on  en=on  dbl_ovrd=off  block_type=register
  Vector Delay : xrbsSSR_Library/Vector Delay  sg_latency=2  infoeditControl=Selection of Reset will increase slice count due to use of real FFs and instead of SRLs  en=off  vectorize_en=off  rst=off  reg_retiming=off  block_type=delay_ssr  dbl_ovrd=off  sg_ssr=16  sg_ssr_prev=16  sg_ssr_name=vect_delay
      settings: SourceProductName=Xilinx SSR Blockset
  Vector Delay1 : xrbsSSR_Library/Vector Delay  sg_latency=2  infoeditControl=Selection of Reset will increase slice count due to use of real FFs and instead of SRLs  en=off  vectorize_en=off  rst=off  reg_retiming=off  block_type=delay_ssr  dbl_ovrd=off  sg_ssr=16  sg_ssr_prev=16  sg_ssr_name=vect_delay
      settings: SourceProductName=Xilinx SSR Blockset
  Vector Slice : xrbsSSR_Library/Vector Slice  nbits=1  sg_ssr=16  sg_ssr_prev=16  boolean_output=on  mode=Upper Bit Location + Width  bit1=0  base1=MSB of Input  bit0=0  base0=LSB of Input  dbl_ovrd=off  block_type=slice_ssr  sg_ssr_name=vect_slice
      settings: SourceProductName=Xilinx SSR Blockset  infoedit="The Vector Slice block supports input of vector types. Extracts a given range of bits from each sample of input vector and presents it at the output.  The output type is ordinarily unsigned with binary point at zero, but can be Boolean when the slice is one bit wide.<br><br>Hardware notes: In hardware this block costs nothing."
  Vector Slice1 : xrbsSSR_Library/Vector Slice  nbits=1  sg_ssr=16  sg_ssr_prev=16  boolean_output=on  mode=Upper Bit Location + Width  bit1=0  base1=MSB of Input  bit0=0  base0=LSB of Input  dbl_ovrd=off  block_type=slice_ssr  sg_ssr_name=vect_slice
      settings: SourceProductName=Xilinx SSR Blockset  infoedit="The Vector Slice block supports input of vector types. Extracts a given range of bits from each sample of input vector and presents it at the output.  The output type is ordinarily unsigned with binary point at zero, but can be Boolean when the slice is one bit wide.<br><br>Hardware notes: In hardware this block costs nothing."
  Vector Slice2 : xrbsSSR_Library/Vector Slice  nbits=1  sg_ssr=16  sg_ssr_prev=16  boolean_output=on  mode=Upper Bit Location + Width  bit1=0  base1=MSB of Input  bit0=0  base0=LSB of Input  dbl_ovrd=off  block_type=slice_ssr  sg_ssr_name=vect_slice
      settings: SourceProductName=Xilinx SSR Blockset  infoedit="The Vector Slice block supports input of vector types. Extracts a given range of bits from each sample of input vector and presents it at the output.  The output type is ordinarily unsigned with binary point at zero, but can be Boolean when the slice is one bit wide.<br><br>Hardware notes: In hardware this block costs nothing."
  Vector to Scalar : xrbsSSR_Library/Vector2Scalar  sg_ssr=16  sg_ssr_prev=16  sg_ssr_name=vect_Vector2Scalar  block_type=vector2scalar_ssr
      settings: SourceProductName=Xilinx SSR Blockset
  Vector to Scalar1 : xrbsSSR_Library/Vector2Scalar  sg_ssr=16  sg_ssr_prev=16  sg_ssr_name=vect_Vector2Scalar  block_type=vector2scalar_ssr
      settings: SourceProductName=Xilinx SSR Blockset
  Vector to Scalar2 : xrbsSSR_Library/Vector2Scalar  sg_ssr=16  sg_ssr_prev=16  sg_ssr_name=vect_Vector2Scalar  block_type=vector2scalar_ssr
      settings: SourceProductName=Xilinx SSR Blockset
  ov : Outport
  wires:
  Register/1 -> ov/1
  A/1 -> Vector Slice/1
  rst/1 -> Register/2
  Constant17/1 -> Register/1
  B/1 -> Vector Slice1/1
  S/1 -> Vector Slice2/1
  Vector Slice/1 -> Vector Delay/1
  Vector Slice1/1 -> Vector Delay1/1
  Vector Delay/1 -> Vector to Scalar/1
  Vector Delay1/1 -> Vector to Scalar1/1
  Vector Slice2/1 -> Vector to Scalar2/1
  Vector to Scalar/1 -> Expression/1
  Vector to Scalar1/1 -> Expression/2
  Vector to Scalar2/1 -> Expression/3
  Expression/1 -> Convert/1
  Convert/1 -> Register/3
